simulink model "varios_tanques_r2019b"  (R2019b)
settings: Solver=ode23tb  StartTime=0.0  StopTime=30.0  RelTol=1e-3  EnableMultiTasking=on
settings Model: Creator=Matias  LastModifiedBy=juanmanueltome
settings DataIOCC: ReturnWorkspaceOutputs=off
settings OptimizationCC: LifeSpan=inf
settings DebuggingCC: SFUnexpectedBacktrackingDiag=warning  SFNoUnconditionalDefaultTransitionDiag=warning  ArithmeticOperatorsInVariantConditions=warning
settings SFSimCC: SimUseLocalCustomCode=off  CustomCodeUndefinedFunction=UseInterfaceOnly
settings RTWCC: RTWUseLocalCustomCode=off
settings CodeAppCC: StateflowObjectComments=on
settings GRTTargetCC: TargetLangStandard=C89/C90 (ANSI)  GeneratePreprocessorConditionals=Disable all
settings ConfigComp: CovMetricSettings=dw  CovHtmlReporting=on  CovSaveCumulativeToWorkspaceVar=on  CovSaveSingleToWorkspaceVar=on  CovExternalEMLEnable=off

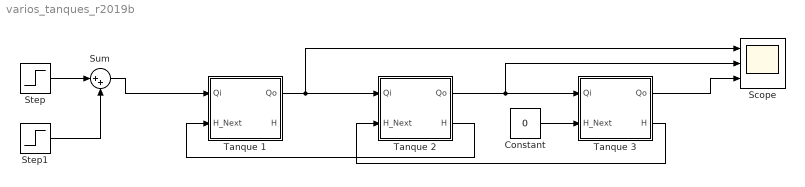
== system varios_tanques_r2019b ==
  Constant : Constant  Value=0
  Scope : Scope  NumInputPorts=3
  Step : Step  SampleTime=0
  Step1 : Step  Time=15  After=-1  SampleTime=0
  Sum : Sum  Inputs=|++
  Tanque 1 : Subsystem
  "Tanque 2 " : Subsystem
  Tanque 3 : Subsystem
  wires:
  Step/1 -> Sum/1
  Sum/1 -> Tanque 1/1("Qi ")
  Step1/1 -> Sum/2
  Tanque 1/1(Qo) -> Scope/1, "Tanque 2 "/1("Qi ")
  "Tanque 2 "/2("H ") -> Tanque 1/2(H_Next)
  "Tanque 2 "/1(Qo) -> Tanque 3/1("Qi "), Scope/2
  Tanque 3/1(Qo) -> Scope/3
  Constant/1 -> Tanque 3/2(H_Next)
  Tanque 3/2("H ") -> "Tanque 2 "/2(H_Next)

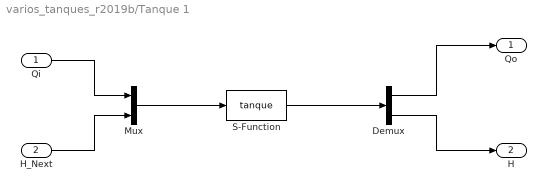
== system varios_tanques_r2019b/Tanque 1 ==
  "Qi " : Inport
  H_Next : Inport  Port=2
  Demux : Demux  Outputs=2
  Mux : Mux  Inputs=2
  S-Function : S-Function  FunctionName=tanque  Parameters=1, 0.75, 1, 0  SFunctionDeploymentMode=off  EnableBusSupport=off
  Qo : Outport
  "H " : Outport  Port=2
  wires:
  Mux/1 -> S-Function/1
  "Qi "/1 -> Mux/1
  H_Next/1 -> Mux/2
  S-Function/1 -> Demux/1
  Demux/2 -> "H "/1
  Demux/1 -> Qo/1

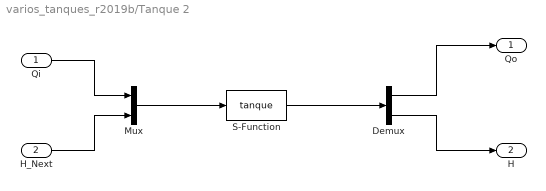
== system varios_tanques_r2019b/Tanque 2  ==
  "Qi " : Inport
  H_Next : Inport  Port=2
  Demux : Demux  Outputs=2
  Mux : Mux  Inputs=2
  S-Function : S-Function  FunctionName=tanque  Parameters=1, 0.75, 1, 0  SFunctionDeploymentMode=off  EnableBusSupport=off
  Qo : Outport
  "H " : Outport  Port=2
  wires:
  Mux/1 -> S-Function/1
  "Qi "/1 -> Mux/1
  H_Next/1 -> Mux/2
  S-Function/1 -> Demux/1
  Demux/2 -> "H "/1
  Demux/1 -> Qo/1

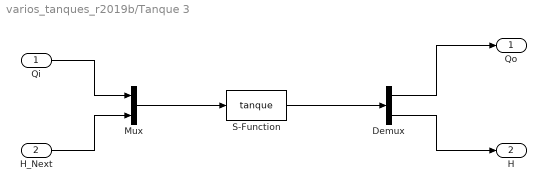
== system varios_tanques_r2019b/Tanque 3 ==
  "Qi " : Inport
  H_Next : Inport  Port=2
  Demux : Demux  Outputs=2
  Mux : Mux  Inputs=2
  S-Function : S-Function  FunctionName=tanque  Parameters=1, 0.75, 1, 0  SFunctionDeploymentMode=off  EnableBusSupport=off
  Qo : Outport
  "H " : Outport  Port=2
  wires:
  Mux/1 -> S-Function/1
  "Qi "/1 -> Mux/1
  H_Next/1 -> Mux/2
  S-Function/1 -> Demux/1
  Demux/2 -> "H "/1
  Demux/1 -> Qo/1
